simulink model "Simulator"  (R2016a)
settings: Solver=VariableStepAuto  StartTime=0.0  StopTime=simulation_time  RelTol=1e-3
InitFcn:
  | Parameters_quadrotor
values from neighbouring files (symbols this model uses):
  delay_altitude = 1    [Parameters_controllers.m]
  delay_attitude = 1    [Parameters_controllers.m]
  delay_mixer = 1    [Parameters_controllers.m]
  delay_position = 1    [Parameters_controllers.m]
  dLMN = [dL_dp  0    0 ... (first row only)    [Parameters_quadrotor.m]
  gravity = 9.81    [Parameters_quadrotor.m]
  inertia_tensor = diag([inertia_xx inertia_yy inertia_zz])    [Parameters_quadrotor.m]
  inertia_tensor_inv = inertia_tensor\eye(3)    [Parameters_quadrotor.m]
  K = [              -Kt,               -Kt,               -Kt,               -Kt ... (first row only)    [Parameters_controllers.m]
  mass = 1.510    (= 1.51)    [Parameters_quadrotor.m]
  mass_matrix = mass * eye(3)    [Parameters_quadrotor.m]
  mass_matrix_inv = (1/mass) * eye(3)    [Parameters_quadrotor.m]
  motor_ome_vs_throttle = [m q]    [Parameters_quadrotor.m]
  motor_tau = 0.055257    [Parameters_quadrotor.m]
  sample_time = 1/sample_frequency    (= 0.01)    [Parameters_controllers.m]
undefined symbols (not defined in the file or in its folder): magnitude, sigbuilder_block
libraries: aerolibutil x2
settings Model: Creator=Mattia  LastModifiedBy=Mattia
settings DataIOCC: SaveFormat=Array

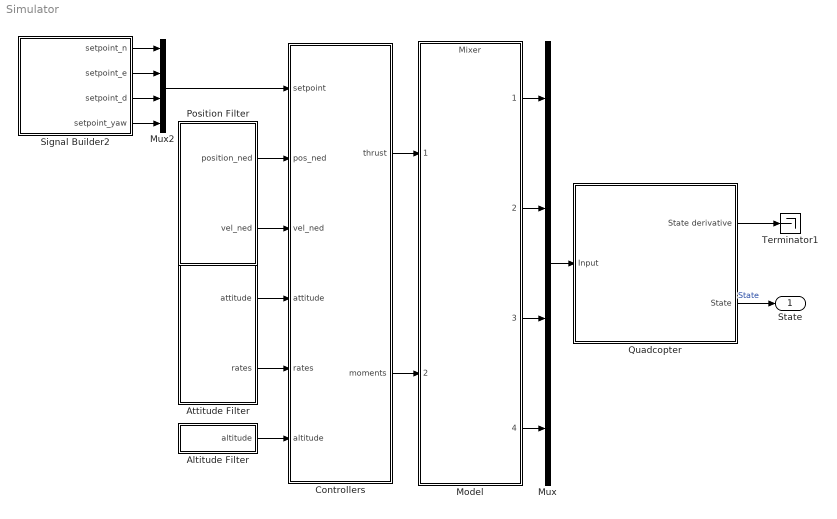
== system Simulator ==
  Altitude Filter : Subsystem
  Attitude Filter : Subsystem
  Controllers : Subsystem
  Model : ModelReference  ModelNameDialog=Mixer.slx  SimulationMode=Normal  ModelReferenceVersion=1.35
  Mux : Mux
  Mux2 : Mux
  Position Filter : Subsystem
  Quadcopter : Subsystem
      mask Display:
      | image(imread('quad.png'))
      | port_label('input',1,'u')
      | port_label('output',1,'Xdot')
      | port_label('output',2,'X')
  Signal Builder2 : Subsystem  Tag=STV Subsys  LoadFcn=sigbuilder_block('load',[6 30 1012.5 447.75 ]);  StartFcn=sigbuilder_block('start');  StopFcn=sigbuilder_block('stop');  ClipboardFcn=sigbuilder_block('clipboard');  mask(Sigbuilder block){}
      mask help: Simulink:masks:SigbuilderBlock_MD
      mask init:
      | if ~strcmp(get_param(bdroot(gcbh),'SimulationStatus'),'stopped') tuvar = sigbuilder_block('maskInit'); end
      settings: CopyFcn=sigbuilder_block('copy');  DeleteFcn=sigbuilder_block('delete');  ModelCloseFcn=sigbuilder_block('modelClose');  PreSaveFcn=sigbuilder_block('preSave');  PauseFcn=sigbuilder_block('pause');  ContinueFcn=sigbuilder_block('continue');  NameChangeFcn=sigbuilder_block('namechange');  OpenFcn=sigbuilder_block('open',[6 30 1012.5 447.75 ]);  CloseFcn=sigbuilder_block('close');
      mask Display: plot(0, 0, 100, 100,[2, 2, 32, 32, 2], [68, 8, 8, 68, 68],[32, 2], [38, 38], [32, 19, 2],[53, 60, 44], [32, 17, 17, 2],[16, 16, 31, 31]);txt = getActiveGroup(gcbh);text(2, 100, txt,'verticalAlignment', 'top');
  Terminator1 : Terminator
  State : Outport
  wires:
  Signal Builder2/2(setpoint_e) -> Mux2/2
  Signal Builder2/3(setpoint_d) -> Mux2/3
  Signal Builder2/4("setpoint_yaw ") -> Mux2/4
  Signal Builder2/1(setpoint_n) -> Mux2/1
  Controllers/2(moments) -> Model/2
  Mux2/1 -> Controllers/1(setpoint)
  Quadcopter/2(State) -> State/1  "State"
  Quadcopter/1(State derivative) -> Terminator1/1
  Attitude Filter/1(attitude) -> Controllers/4(attitude)
  Altitude Filter/1(altitude) -> Controllers/6(altitude)
  Mux/1 -> Quadcopter/1(Input)
  Model/1 -> Mux/1
  Model/2 -> Mux/2
  Model/3 -> Mux/3
  Model/4 -> Mux/4
  Controllers/1(thrust) -> Model/1
  Attitude Filter/2(rates) -> Controllers/5(rates)
  Position Filter/1(position_ned) -> Controllers/2(pos_ned)
  Position Filter/2(vel_ned) -> Controllers/3(vel_ned)

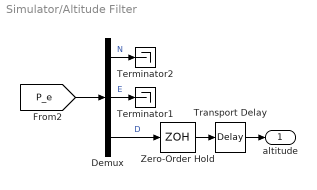
== system Simulator/Altitude Filter ==
  Demux : Demux  Outputs=3
  Terminator1 : Terminator
  Terminator2 : Terminator
  Transport Delay : TransportDelay  DelayTime=delay_altitude * sample_time
  Zero-Order Hold : ZeroOrderHold  SampleTime=sample_time
  altitude : Outport
  wires:
  Demux/2 -> Terminator1/1  "E"
  [P_e] -> Demux/1
  Demux/1 -> Terminator2/1  "N"
  Zero-Order Hold/1 -> Transport Delay/1
  Demux/3 -> Zero-Order Hold/1  "D"
  Transport Delay/1 -> altitude/1

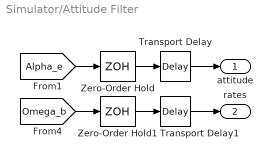
== system Simulator/Attitude Filter ==
  Transport Delay : TransportDelay  DelayTime=delay_attitude * sample_time
  Transport Delay1 : TransportDelay  DelayTime=delay_attitude * sample_time
  Zero-Order Hold : ZeroOrderHold  SampleTime=sample_time
  Zero-Order Hold1 : ZeroOrderHold  SampleTime=sample_time
  attitude : Outport  PortDimensions=3
  rates : Outport  Port=2  PortDimensions=3
  wires:
  [Omega_b] -> Zero-Order Hold1/1
  [Alpha_e] -> Zero-Order Hold/1
  Zero-Order Hold1/1 -> Transport Delay1/1
  Zero-Order Hold/1 -> Transport Delay/1
  Transport Delay1/1 -> rates/1
  Transport Delay/1 -> attitude/1

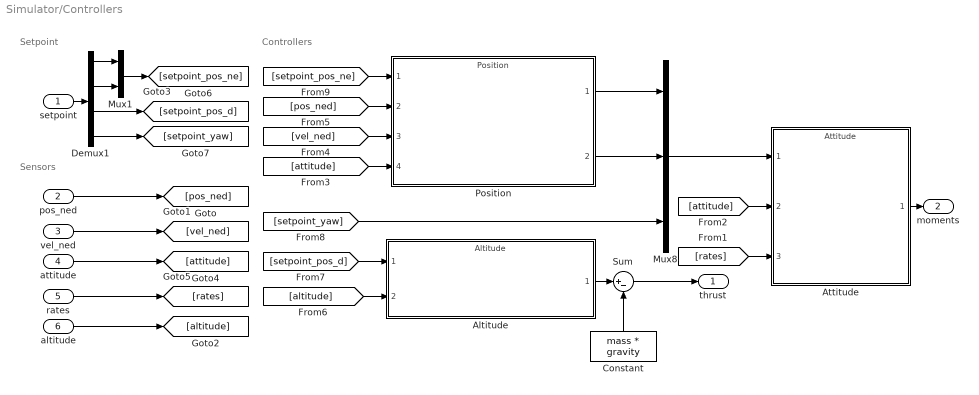
== system Simulator/Controllers ==
  note: Sensors
  note: Setpoint
  note: Controllers
  setpoint : Inport  PortDimensions=4
  pos_ned : Inport  Port=2  PortDimensions=2
  vel_ned : Inport  Port=3  PortDimensions=2
  attitude : Inport  Port=4  PortDimensions=3
  rates : Inport  Port=5  PortDimensions=3
  altitude : Inport  Port=6  PortDimensions=1
  Altitude : ModelReference  ModelNameDialog=Altitude.slx  SimulationMode=Normal  ModelReferenceVersion=1.115
  Attitude : ModelReference  ModelNameDialog=Attitude.slx  SimulationMode=Normal  ModelReferenceVersion=1.162
  Constant : Constant  Value=mass * gravity
  Demux1 : Demux
  Mux1 : Mux  Inputs=2
  Mux8 : Mux  Inputs=3
  Position : ModelReference  ModelNameDialog=Position.slx  SimulationMode=Normal  ModelReferenceVersion=1.254
  Sum : Sum  Inputs=|+-
  thrust : Outport
  moments : Outport  Port=2  PortDimensions=3
  wires:
  setpoint/1 -> Demux1/1
  [attitude] -> Attitude/2
  Demux1/4 -> [setpoint_yaw]
  Demux1/2 -> Mux1/2
  Demux1/1 -> Mux1/1
  Attitude/1 -> moments/1
  [pos_ned] -> Position/2
  Mux8/1 -> Attitude/1
  [rates] -> Attitude/3
  Altitude/1 -> Sum/1
  Constant/1 -> Sum/2
  [setpoint_yaw] -> Mux8/3
  attitude/1 -> [attitude]
  altitude/1 -> [altitude]
  Demux1/3 -> [setpoint_pos_d]
  Mux1/1 -> [setpoint_pos_ne]
  [setpoint_pos_d] -> Altitude/1
  [setpoint_pos_ne] -> Position/1
  pos_ned/1 -> [pos_ned]
  vel_ned/1 -> [vel_ned]
  rates/1 -> [rates]
  [attitude] -> Position/4
  [altitude] -> Altitude/2
  Sum/1 -> thrust/1
  [vel_ned] -> Position/3
  Position/1 -> Mux8/1
  Position/2 -> Mux8/2

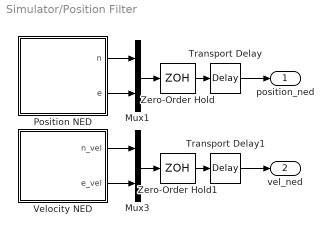
== system Simulator/Position Filter ==
  Mux1 : Mux  Inputs=2
  Mux3 : Mux  Inputs=2
  Position NED : Subsystem
  Transport Delay : TransportDelay  DelayTime=delay_position * sample_time
  Transport Delay1 : TransportDelay  DelayTime=delay_position * sample_time
  Velocity NED : Subsystem
  Zero-Order Hold : ZeroOrderHold  SampleTime=sample_time
  Zero-Order Hold1 : ZeroOrderHold  SampleTime=sample_time
  position_ned : Outport  PortDimensions=2
  vel_ned : Outport  Port=2  PortDimensions=2
  wires:
  Position NED/2(e) -> Mux1/2
  Velocity NED/2(e_vel) -> Mux3/2
  Velocity NED/1(n_vel) -> Mux3/1
  Position NED/1(n) -> Mux1/1
  Zero-Order Hold/1 -> Transport Delay/1
  Mux1/1 -> Zero-Order Hold/1
  Transport Delay/1 -> position_ned/1
  Zero-Order Hold1/1 -> Transport Delay1/1
  Mux3/1 -> Zero-Order Hold1/1
  Transport Delay1/1 -> vel_ned/1

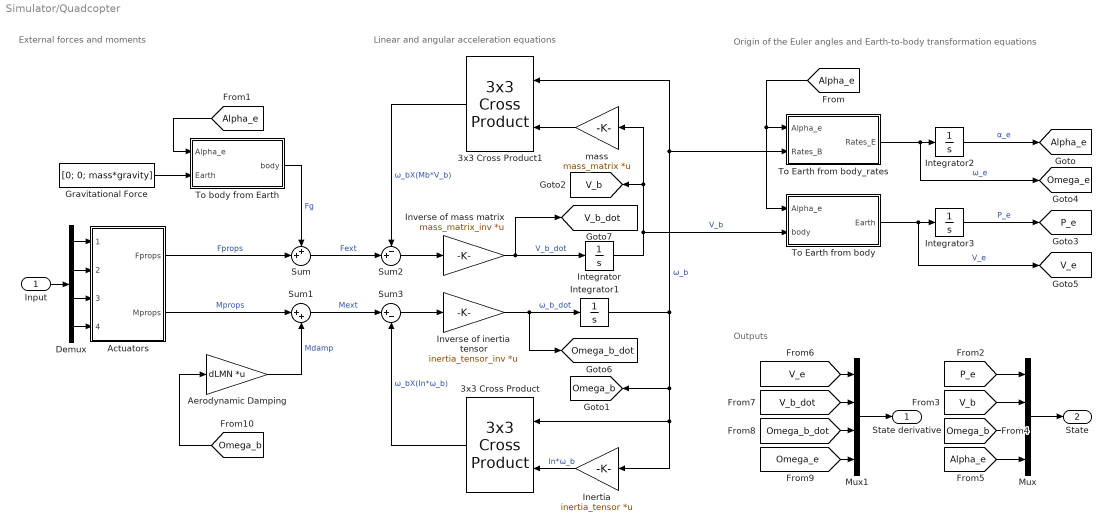
== system Simulator/Quadcopter ==
  note: Outputs
  note: Origin of the Euler angles and Earth-to-body transformation equations
  note: Linear and angular acceleration equations
  note: External forces and moments
  Input : Inport
  3x3 Cross Product : aerolibutil/3x3 Cross Product
  3x3 Cross Product1 : aerolibutil/3x3 Cross Product
  Actuators : Subsystem
  Aerodynamic Damping : Gain  Gain=dLMN  Multiplication=Matrix(K*u)
  Demux : Demux
  Gravitational Force : Constant  Value=[0; 0; mass*gravity]
  Inertia : Gain  Gain=inertia_tensor  Multiplication=Matrix(K*u)
  Integrator{,1..3} (4 alike) : Integrator  InitialCondition=[0; 0; 0]
  Inverse of inertia tensor : Gain  Gain=inertia_tensor_inv  Multiplication=Matrix(K*u)
  Inverse of mass matrix : Gain  Gain=mass_matrix_inv  Multiplication=Matrix(K*u)
  Mux : Mux
  Mux1 : Mux
  Sum : Sum  Inputs=++|
  Sum1 : Sum  Inputs=|++
  Sum2 : Sum  Inputs=-+|
  Sum3 : Sum  Inputs=|+-
  To Earth from body : MATLAB Function  TreatAsAtomicUnit=on
  To Earth from body_rates : MATLAB Function  TreatAsAtomicUnit=on
  To body from Earth : MATLAB Function  TreatAsAtomicUnit=on
  mass : Gain  Gain=mass_matrix  Multiplication=Matrix(K*u)
  State derivative : Outport
  State : Outport  Port=2
  tag scope: Alpha_e=global, Omega_b=global, Omega_b_dot=global, Omega_e=global, P_e=global, V_b=global, V_b_dot=global, V_e=global
  wires:
  To Earth from body_rates/1(Rates_E) -> Integrator2/1, [Omega_e]  "ω_e"
  [P_e] -> Mux/1
  Actuators/2(Mprops) -> Sum1/1  "Mprops"
  Input/1 -> Demux/1
  3x3 Cross Product/1 -> Sum3/2  "ω_bX(In*ω_b)"
  [V_b_dot] -> Mux1/2
  Mux/1 -> State/1
  Mux1/1 -> State derivative/1
  [V_b] -> Mux/2
  [Alpha_e] -> Mux/4
  [Omega_b] -> Mux/3
  Demux/4 -> Actuators/4(Th4 [%])
  [Omega_e] -> Mux1/4
  [Omega_b_dot] -> Mux1/3
  [V_e] -> Mux1/1
  Demux/3 -> Actuators/3(Th3 [%])
  Inverse of mass matrix/1 -> Integrator/1, [V_b_dot]  "V_b_dot"
  Integrator/1 -> To Earth from body/2(body), mass/1, [V_b]  "V_b"
  [Alpha_e] -> To Earth from body/1(Alpha_e), To Earth from body_rates/1(Alpha_e)
  Integrator1/1 -> To Earth from body_rates/2(Rates_B), 3x3 Cross Product1/1, 3x3 Cross Product/1, Inertia/1, [Omega_b]  "ω_b"
  Sum3/1 -> Inverse of inertia tensor/1
  Sum2/1 -> Inverse of mass matrix/1
  mass/1 -> 3x3 Cross Product1/2
  Sum/1 -> Sum2/2  "Fext"
  Sum1/1 -> Sum3/1  "Mext"
  Demux/1 -> Actuators/1(Th1 [%])
  Demux/2 -> Actuators/2(Th2 [%])
  Inverse of inertia tensor/1 -> Integrator1/1, [Omega_b_dot]  "ω_b_dot"
  3x3 Cross Product1/1 -> Sum2/1  "ω_bX(Mb*V_b)"
  Integrator2/1 -> [Alpha_e]  "α_e"
  Aerodynamic Damping/1 -> Sum1/2  "Mdamp"
  Actuators/1(Fprops) -> Sum/2  "Fprops"
  Integrator3/1 -> [P_e]  "P_e"
  Inertia/1 -> 3x3 Cross Product/2  "In*ω_b"
  [Omega_b] -> Aerodynamic Damping/1
  To Earth from body/1(Earth) -> [V_e], Integrator3/1  "V_e"
  To body from Earth/1(body) -> Sum/1  "Fg"
  Gravitational Force/1 -> To body from Earth/2(Earth)
  [Alpha_e] -> To body from Earth/1(Alpha_e)

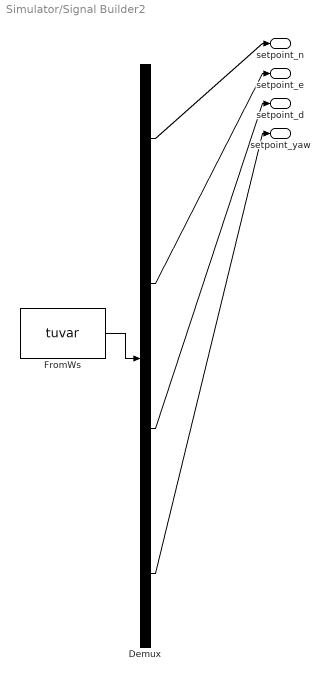
== system Simulator/Signal Builder2 ==
  Demux : Demux  Tag=STV Demux
  FromWs : FromWorkspace  Tag=STV FromWs  VariableName=tuvar  SampleTime=0
      SigBuilderData=|
      | common.afterFinalStr = 'Extrapolate'
      | common.sampleTime = 0
      | dataSet(1).timeRange = [0 50]
      | dataSet(1).name = 'setpoint'
      | dataSet(2).timeRange = [0 50]
      | dataSet(2).name = 'Set-point_2'
      | sbobj.Groups(1).Name = 'setpoint'
      | sbobj.Groups(1).Signals(1).Name = 'setpoint_n'
      | sbobj.Groups(1).Signals(1).XData = [0 10 10 15 30 35 50]
      | sbobj.Groups(1).Signals(1).YData = [0 -0.005 0.005 1 1 0.02 0]
      | sbobj.Groups(1).Signals(2).Name = 'setpoint_e'
      | sbobj.Groups(1).Signals(2).XData = [0 50]
      | sbobj.Groups(1).Signals(2).YData = [0 0]
      | sbobj.Groups(1).Signals(3).Name = 'setpoint_d'
      | sbobj.Groups(1).Signals(3).XData = [0 50]
      | sbobj.Groups(1).Signals(3).YData = [-1 -1]
      | sbobj.Groups(1).Signals(4).Name = 'setpoint_yaw '
      | sbobj.Groups(1).Signals(4).XData = [0 10 40 50]
      | sbobj.Groups(1).Signals(4).YData = [0 0 0 0]
      | sbobj.Groups(1).TimeRange = [0 50]
      | sbobj.Groups(2).Name = 'Set-point_2'
      | sbobj.Groups(2).Signals(1).Name = 'setpoint_n'
      | sbobj.Groups(2).Signals(1).XData = [0 10 45 45.05 50]
      | sbobj.Groups(2).Signals(1).YData = [0 0 1 0 0]
      | sbobj.Groups(2).Signals(2).Name = 'setpoint_e'
      | sbobj.Groups(2).Signals(2).XData = [0 10 50]
      | sbobj.Groups(2).Signals(2).YData = [0 0 0]
      | sbobj.Groups(2).Signals(3).Name = 'setpoint_d'
      | sbobj.Groups(2).Signals(3).XData = [0 50]
      | sbobj.Groups(2).Signals(3).YData = [-2 -2]
      | sbobj.Groups(2).Signals(4).Name = 'setpoint_yaw '
      | sbobj.Groups(2).Signals(4).XData = [0 10 40 50]
      | sbobj.Groups(2).Signals(4).YData = [0 0 0 0]
      | sbobj.Groups(2).TimeRange = [0 50]
  setpoint_n : Outport  Tag=STV Outport
  setpoint_e : Outport  Tag=STV Outport  Port=2
  setpoint_d : Outport  Tag=STV Outport  Port=3
  "setpoint_yaw " : Outport  Tag=STV Outport  Port=4
  wires:
  FromWs/1 -> Demux/1
  Demux/1 -> setpoint_n/1
  Demux/2 -> setpoint_e/1
  Demux/3 -> setpoint_d/1
  Demux/4 -> "setpoint_yaw "/1

== system Simulator/Position Filter/Position NED ==
  Demux : Demux  Outputs=3
  Terminator : Terminator
  n : Outport
  e : Outport  Port=2
  wires:
  Demux/1 -> n/1  "n"
  Demux/3 -> Terminator/1  "d"
  [P_e] -> Demux/1
  Demux/2 -> e/1  "e"

== system Simulator/Position Filter/Velocity NED ==
  Demux : Demux  Outputs=3
  Terminator : Terminator
  n_vel : Outport
  e_vel : Outport  Port=2
  wires:
  Demux/2 -> e_vel/1  "e"
  [V_e] -> Demux/1
  Demux/3 -> Terminator/1  "d"
  Demux/1 -> n_vel/1  "n_vel"

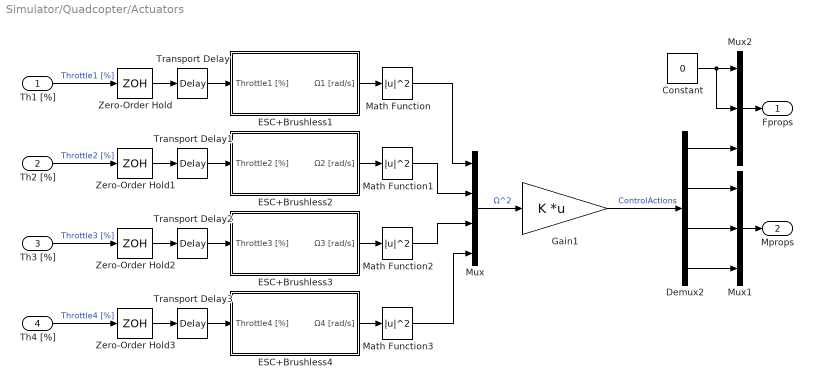
== system Simulator/Quadcopter/Actuators ==
  Th1 [%] : Inport
  Th2 [%] : Inport  Port=2
  Th3 [%] : Inport  Port=3
  Th4 [%] : Inport  Port=4
  Constant : Constant  Value=0
  Demux2 : Demux
  ESC+Brushless1 : Subsystem
  ESC+Brushless2 : Subsystem
  ESC+Brushless3 : Subsystem
  ESC+Brushless4 : Subsystem
  Gain1 : Gain  Gain=K  Multiplication=Matrix(K*u)
  Math Function{,1..3} (4 alike) : Math  Operator=magnitude^2  SaturateOnIntegerOverflow=on
  Mux : Mux
  Mux1 : Mux  Inputs=3
  Mux2 : Mux  Inputs=3
  Transport Delay{,1..3} (4 alike) : TransportDelay  DelayTime=delay_mixer * sample_time
  Zero-Order Hold{,1..3} (4 alike) : ZeroOrderHold  SampleTime=sample_time
  Fprops : Outport
  Mprops : Outport  Port=2
  wires:
  Gain1/1 -> Demux2/1  "ControlActions"
  Th1 [%]/1 -> Zero-Order Hold/1  "Throttle1 [%]"
  Th2 [%]/1 -> Zero-Order Hold1/1  "Throttle2 [%]"
  Th4 [%]/1 -> Zero-Order Hold3/1  "Throttle4 [%]"
  Th3 [%]/1 -> Zero-Order Hold2/1  "Throttle3 [%]"
  ESC+Brushless1/1(Ω1 [rad/s]) -> Math Function/1
  ESC+Brushless2/1(Ω2 [rad/s]) -> Math Function1/1
  ESC+Brushless3/1(Ω3 [rad/s]) -> Math Function2/1
  ESC+Brushless4/1(Ω4 [rad/s]) -> Math Function3/1
  Mux/1 -> Gain1/1  "Ω^2"
  Math Function/1 -> Mux/1
  Math Function1/1 -> Mux/2
  Math Function2/1 -> Mux/3
  Math Function3/1 -> Mux/4
  Mux1/1 -> Mprops/1
  Demux2/2 -> Mux1/1
  Demux2/3 -> Mux1/2
  Demux2/4 -> Mux1/3
  Demux2/1 -> Mux2/3
  Constant/1 -> Mux2/2, Mux2/1
  Mux2/1 -> Fprops/1
  Transport Delay/1 -> ESC+Brushless1/1(Throttle1 [%])
  Transport Delay1/1 -> ESC+Brushless2/1(Throttle2 [%])
  Transport Delay3/1 -> ESC+Brushless4/1(Throttle4 [%])
  Transport Delay2/1 -> ESC+Brushless3/1(Throttle3 [%])
  Zero-Order Hold/1 -> Transport Delay/1
  Zero-Order Hold1/1 -> Transport Delay1/1
  Zero-Order Hold2/1 -> Transport Delay2/1
  Zero-Order Hold3/1 -> Transport Delay3/1

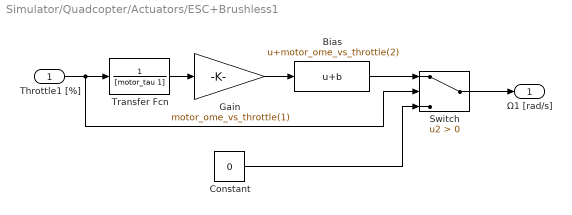
== system Simulator/Quadcopter/Actuators/ESC+Brushless1 ==
  Throttle1 [%] : Inport
  Bias : Bias  Bias=motor_ome_vs_throttle(2)
  Constant : Constant  Value=0
  Gain : Gain  Gain=motor_ome_vs_throttle(1)
  Switch : Switch  Criteria=u2 > Threshold
  Transfer Fcn : TransferFcn  Denominator=[motor_tau 1]
  Ω1 [rad/s] : Outport
  wires:
  Gain/1 -> Bias/1
  Bias/1 -> Switch/1
  Constant/1 -> Switch/3
  Switch/1 -> Ω1 [rad/s]/1
  Throttle1 [%]/1 -> Transfer Fcn/1, Switch/2
  Transfer Fcn/1 -> Gain/1

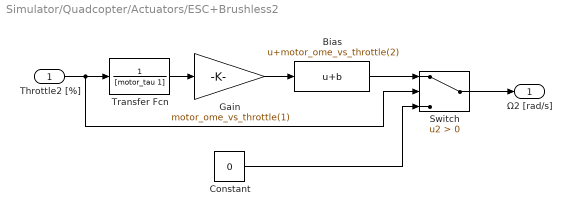
== system Simulator/Quadcopter/Actuators/ESC+Brushless2 ==
  Throttle2 [%] : Inport
  Bias : Bias  Bias=motor_ome_vs_throttle(2)
  Constant : Constant  Value=0
  Gain : Gain  Gain=motor_ome_vs_throttle(1)
  Switch : Switch  Criteria=u2 > Threshold
  Transfer Fcn : TransferFcn  Denominator=[motor_tau 1]
  Ω2 [rad/s] : Outport
  wires:
  Gain/1 -> Bias/1
  Bias/1 -> Switch/1
  Constant/1 -> Switch/3
  Switch/1 -> Ω2 [rad/s]/1
  Throttle2 [%]/1 -> Transfer Fcn/1, Switch/2
  Transfer Fcn/1 -> Gain/1

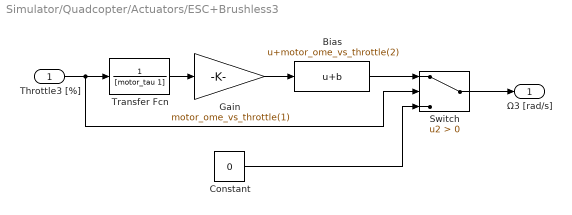
== system Simulator/Quadcopter/Actuators/ESC+Brushless3 ==
  Throttle3 [%] : Inport
  Bias : Bias  Bias=motor_ome_vs_throttle(2)
  Constant : Constant  Value=0
  Gain : Gain  Gain=motor_ome_vs_throttle(1)
  Switch : Switch  Criteria=u2 > Threshold
  Transfer Fcn : TransferFcn  Denominator=[motor_tau 1]
  Ω3 [rad/s] : Outport
  wires:
  Gain/1 -> Bias/1
  Bias/1 -> Switch/1
  Constant/1 -> Switch/3
  Switch/1 -> Ω3 [rad/s]/1
  Throttle3 [%]/1 -> Transfer Fcn/1, Switch/2
  Transfer Fcn/1 -> Gain/1

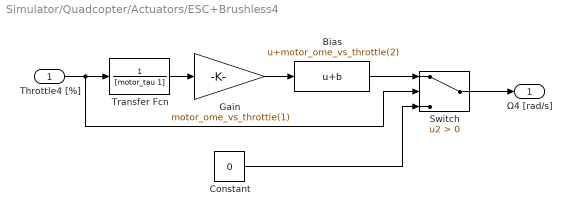
== system Simulator/Quadcopter/Actuators/ESC+Brushless4 ==
  Throttle4 [%] : Inport
  Bias : Bias  Bias=motor_ome_vs_throttle(2)
  Constant : Constant  Value=0
  Gain : Gain  Gain=motor_ome_vs_throttle(1)
  Switch : Switch  Criteria=u2 > Threshold
  Transfer Fcn : TransferFcn  Denominator=[motor_tau 1]
  Ω4 [rad/s] : Outport
  wires:
  Gain/1 -> Bias/1
  Bias/1 -> Switch/1
  Constant/1 -> Switch/3
  Switch/1 -> Ω4 [rad/s]/1
  Throttle4 [%]/1 -> Transfer Fcn/1, Switch/2
  Transfer Fcn/1 -> Gain/1

== matlab function Simulator/Quadcopter/To body from Earth ==
  data: Alpha_e input; Earth input; body output
 function body = Tbe(Alpha_e, Earth)
%#codegen
phi = Alpha_e(1);
theta = Alpha_e(2);
psi = Alpha_e(3);

Sphi = sin(phi);
Cphi = cos(phi);
Stheta = sin(theta);
Ctheta = cos(theta);
Spsi = sin(psi);
Cpsi = cos(psi);

TBE = [        Ctheta*Cpsi               Ctheta*Spsi          -Stheta    ;
       Sphi*Stheta*Cpsi-Cphi*Spsi Sphi*Stheta*Spsi+Cphi*Cpsi Sphi*Ctheta ;
       Cphi*Stheta*Cpsi+Sphi*Spsi Cphi*Stheta*Spsi-Sphi*Cpsi Cphi*Ctheta];

body = TBE* Earth;

== matlab function Simulator/Quadcopter/To Earth from body ==
  data: Alpha_e input; Earth output; body input
 function Earth = Tbet(Alpha_e, body)
%#codegen
phi = Alpha_e(1);
theta = Alpha_e(2);
psi = Alpha_e(3);

Sphi = sin(phi);
Cphi = cos(phi);
Stheta = sin(theta);
Ctheta = cos(theta);
Spsi = sin(psi);
Cpsi = cos(psi);

TBE = [        Ctheta*Cpsi               Ctheta*Spsi          -Stheta    ;
       Sphi*Stheta*Cpsi-Cphi*Spsi Sphi*Stheta*Spsi+Cphi*Cpsi Sphi*Ctheta ;
       Cphi*Stheta*Cpsi+Sphi*Spsi Cphi*Stheta*Spsi-Sphi*Cpsi Cphi*Ctheta];
TEB = TBE';

Earth = TEB* body;

== matlab function Simulator/Quadcopter/To Earth from body_rates ==
  data: Alpha_e input; Rates_B input; Rates_E output
 function Rates_E = Einv(Alpha_e, Rates_B)
%#codegen
phi = Alpha_e(1);
theta = Alpha_e(2);

Sphi = sin(phi);
Cphi = cos(phi);
Ctheta = cos(theta);
Ttheta = tan(theta);

Einv = [1   Sphi*Ttheta    Cphi*Ttheta ;
        0       Cphi          -Sphi    ;
        0   Sphi/Ctheta    Cphi/Ctheta];

Rates_E = Einv* Rates_B;
